simulink model "Roll_Reduced_Model_R2023b"  (R2023b)
settings: Solver=VariableStepAuto  StartTime=0.0  StopTime=10.0  RelTol=1e-3
PreLoadFcn:
  | MyParameters
values from neighbouring files (symbols this model uses):
  b = 0    [MyParameters.m]
  CurrThrust = 50    [MyParameters.m]
  g = 9.81    [MyParameters.m]
  Jpitch = 0.076089    [MyParameters.m]
  Jroll = 0.0520129    [MyParameters.m]
  Lp = 0.24    [MyParameters.m]
  Lr = 0.24    [MyParameters.m]
  mp = 2.464    [MyParameters.m]
  mr = 2    [MyParameters.m]
  rp = 0.107654    [MyParameters.m]
  rr = 0.072538    [MyParameters.m]
libraries: slpidlib x4, simulink x2
settings Model: Creator=user  LastModifiedBy=user
settings SolverCC: AlgebraicLoopSolver=TrustRegion

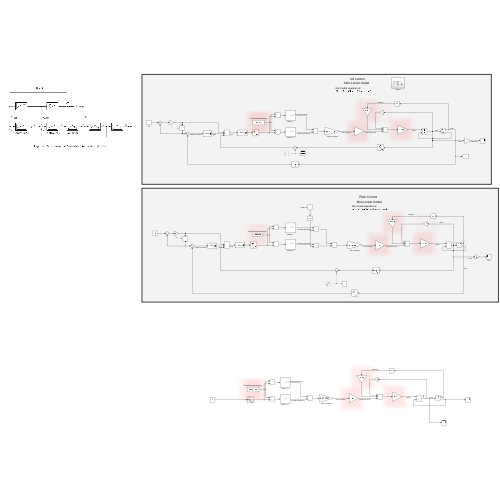
[thumbnail: Simulink's stored preview of the top-level diagram]
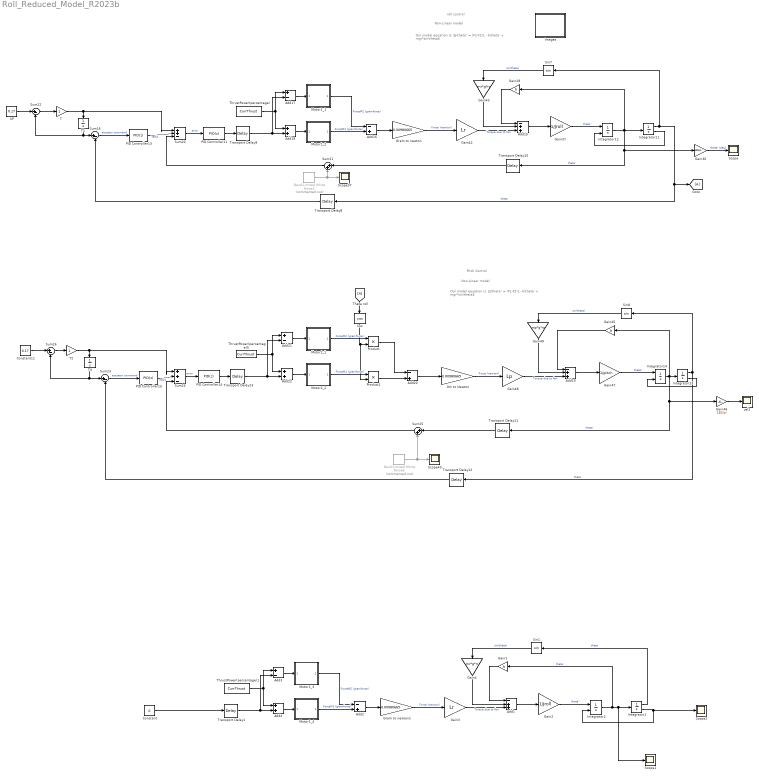
== system Roll_Reduced_Model_R2023b ==
  note: Our model equation is:
      | $J\theta'' = (F1-F2)L - b\theta' + mgr*sin\theta$
  note: Our model equation is:
      | $J\theta'' = (F1-F2)L - b\theta' + mgr*sin\theta$
  note: Non-Linear model
  note: Pitch Control
  note: Non-Linear model
  note: roll control
  Add1 : Sum  Inputs=-++
  Add15 : Sum  Inputs=-++
  Add16 : Sum  Inputs=-+
  Add17 : Sum  Inputs=+-
  Add18 : Sum
  Add19 : Sum  Inputs=-++
  Add2 : Sum  Inputs=-+
  Add20 : Sum  Inputs=-+
  Add21 : Sum  Inputs=+-
  Add22 : Sum
  Add3 : Sum  Inputs=+-
  Add4 : Sum
  Band-Limited White Noise3 : simulink/Sources/Band-Limited White Noise  Commented=on  Cov=0.000005  Ts=0.0225  seed=[23341]
  Band-Limited White Noise5 : simulink/Sources/Band-Limited White Noise  Commented=on  Cov=0.000005  Ts=0.0225  seed=[23341]
  Constant : Constant  Value=0
  Constant11 : Constant  Value=0.17
  Cos : Trigonometry  Operator=cos
  Gain1 : Gain  Gain=b
  Gain2 : Gain  Gain=1/Jroll
  Gain28 : Gain  Gain=b
  Gain3 : Gain  Gain=Lr
  Gain36 : Gain  Gain=180/pi
  Gain37 : Gain  Gain=1/Jroll
  Gain4 : Gain  Gain=mr*g*rr
  Gain42 : Gain  Gain=Lr
  Gain43 : Gain  Gain=mr*g*rr
  Gain45 : Gain  Gain=b
  Gain46 : Gain  Gain=180/pi
  Gain47 : Gain  Gain=1/Jpitch
  Gain48 : Gain  Gain=Lp
  Gain49 : Gain  Gain=mp*g*rp
  Gm to Newton : Gain  Gain=0.00980665
  Goto : Goto
  Gram to newton : Gain  Gain=0.00980665
  Gram to newton1 : Gain  Gain=0.00980665
  Images : Subsystem
  Integrator1 : Integrator  LimitOutput=on  UpperSaturationLimit=0.7  LowerSaturationLimit=-0.7  ShowSaturationPort=on
  Integrator11 : Integrator  LimitOutput=on  UpperSaturationLimit=0.7  LowerSaturationLimit=-0.7  ShowSaturationPort=on
  Integrator12 : Integrator  ExternalReset=level hold
  Integrator13 : Integrator  LimitOutput=on  UpperSaturationLimit=0.7  LowerSaturationLimit=-0.7  ShowSaturationPort=on
  Integrator14 : Integrator  ExternalReset=level hold
  Integrator2 : Integrator  ExternalReset=level hold
  Motor1_1 : Subsystem
      mask Display: image('2200kv.jpg');
  Motor1_2 : Subsystem
      mask Display: image('2200kv.jpg');
  Motor1_3 : Subsystem
      mask Display: image('2200kv.jpg');
  Motor1_4 : Subsystem
      mask Display: image('2200kv.jpg');
  Motor2_1 : Subsystem
      mask Display: image('2200kv.jpg');
  Motor2_2 : Subsystem
      mask Display: image('2200kv.jpg');
  PID Controller11 : slpidlib/PID Controller  Controller=PID  Form=Parallel  TimeDomain=Discrete-time  UseExternalTs=off  SampleTime=0.005  IntegratorMethod=Forward Euler  FilterMethod=Forward Euler  ControllerParametersSource=internal  P=4.5  I=60  UseKiTs=off  D=1.2  N=10  UseFilter=on  TunerSelectOption=Transfer Function Based (PID Tuner App)  InitialConditionSource=internal  InitialConditionForIntegrator=0  InitialConditionForFilter=0  DifferentiatorICPrevScaledInput=0  ExternalReset=none  TrackingMode=off  Kt=1  LimitOutput=on  SatLimitsSource=internal  UpperSaturationLimit=40  LowerSaturationLimit=-40  LinearizeAsGain=on  AntiWindupMode=clamping  Kb=1  LimitIntegrator=off  UpperIntegratorSaturationLimit=inf  LowerIntegratorSaturationLimit=-inf  POutMin=[]  POutMax=[]  IOutMin=[]  IOutMax=[]  DOutMin=[]  DOutMax=[]  NOutMin=[]  NOutMax=[]  SumOutMin=[]  SumOutMax=[]  SaturationOutMin=[]  SaturationOutMax=[]  PParamMin=[]  PParamMax=[]  IParamMin=[]  IParamMax=[]  DParamMin=[]  DParamMax=[]  NParamMin=[]  NParamMax=[]  KbParamMin=[]  KbParamMax=[]  KtParamMin=[]  KtParamMax=[]  KbOutMin=[]  KbOutMax=[]  KtOutMin=[]  KtOutMax=[]  IntegratorOutMin=[]  IntegratorOutMax=[]  FilterOutMin=[]  FilterOutMax=[]  SumI1OutMin=[]  SumI1OutMax=[]  SumI2OutMin=[]  SumI2OutMax=[]  SumI3OutMin=[]  SumI3OutMax=[]  SumI4OutMin=[]  SumI4OutMax=[]  SumDOutMin=[]  SumDOutMax=[]  DifferentiatorOutMin=[]  DifferentiatorOutMax=[]  FilterDiffOutCoefMin=[]  FilterDiffOutCoefMax=[]  ReciprocalOutMin=[]  ReciprocalOutMax=[]  SumDenOutMin=[]  SumDenOutMax=[]  SumNumOutMin=[]  SumNumOutMax=[]  DivideOutMin=[]  DivideOutMax=[]  UdiffTsProdOutMin=[]  UdiffTsProdOutMax=[]  NTsProdOutMin=[]  NTsProdOutMax=[]  UintegralTsProdOutMin=[]  UintegralTsProdOutMax=[]  UngainTsProdOutMin=[]  UngainTsProdOutMax=[]  ClampingZeroOutDataTypeStr=Inherit: Inherit via back propagation  ClampingZeroOutMin=[]  ClampingZeroOutMax=[]  FilterDenConstantOutDataTypeStr=Inherit: Inherit via back propagation  FilterDenConstantOutMin=[]  FilterDenConstantOutMax=[]  PCopyOutDataTypeStr=Inherit: Inherit via back propagation  PCopyOutMin=[]  PCopyOutMax=[]  NCopyOutDataTypeStr=Inherit: Inherit via back propagation  NCopyOutMin=[]  NCopyOutMax=[]  IntegratorContinuousStateAttributes=''  IntegratorStateMustResolveToSignalObject=off  IntegratorRTWStateStorageClass=Auto  FilterContinuousStateAttributes=''  FilterStateMustResolveToSignalObject=off  FilterRTWStateStorageClass=Auto  ParallelPVariant=InternalParameters  IdealPVariant=Disabled  IVariant=InternalParameters  DVariant=InternalParameters  IntegratorVariant=Discrete  SatVariant=Enabled  AWVariant=DiscClampingParallel  PCopyVariant=Disabled  TRVariant=Disabled  FdbkBlocksVariant=Forward  IdealPFdbkVariant=Disabled  SatFdbkVariant=Disabled  DerivativeFilterVariant=ForwardEulerFilter  NVariant=InternalParameters  NCopyVariant=Disabled  FilterICVariant=InternalICsFilter  IntegratorICVariant=InternalICs  ExternalResetVariant=Disabled  TRSumVariant=Passthrough  SumFdbkVariant=Disabled  SumVariant=Sum_PID  TsampFilterVariant=InternalTs  TsampNgainVariant=Passthrough  TsampIntegralVariant=Disabled_SignalSpec  ExternalSaturationOutDataTypeStr=Inherit: Same as second input
  PID Controller13 : slpidlib/PID Controller  Controller=PID  Form=Parallel  TimeDomain=Discrete-time  UseExternalTs=off  SampleTime=0.005  IntegratorMethod=Forward Euler  FilterMethod=Forward Euler  ControllerParametersSource=internal  P=1.2  I=0  UseKiTs=off  D=0  N=100  UseFilter=on  TunerSelectOption=Transfer Function Based (PID Tuner App)  InitialConditionSource=internal  InitialConditionForIntegrator=0  InitialConditionForFilter=0  DifferentiatorICPrevScaledInput=0  ExternalReset=none  TrackingMode=off  Kt=1  LimitOutput=on  SatLimitsSource=internal  UpperSaturationLimit=30  LowerSaturationLimit=-30  LinearizeAsGain=on  AntiWindupMode=clamping  Kb=1  LimitIntegrator=off  UpperIntegratorSaturationLimit=inf  LowerIntegratorSaturationLimit=-inf  POutMin=[]  POutMax=[]  IOutMin=[]  IOutMax=[]  DOutMin=[]  DOutMax=[]  NOutMin=[]  NOutMax=[]  SumOutMin=[]  SumOutMax=[]  SaturationOutMin=[]  SaturationOutMax=[]  PParamMin=[]  PParamMax=[]  IParamMin=[]  IParamMax=[]  DParamMin=[]  DParamMax=[]  NParamMin=[]  NParamMax=[]  KbParamMin=[]  KbParamMax=[]  KtParamMin=[]  KtParamMax=[]  KbOutMin=[]  KbOutMax=[]  KtOutMin=[]  KtOutMax=[]  IntegratorOutMin=[]  IntegratorOutMax=[]  FilterOutMin=[]  FilterOutMax=[]  SumI1OutMin=[]  SumI1OutMax=[]  SumI2OutMin=[]  SumI2OutMax=[]  SumI3OutMin=[]  SumI3OutMax=[]  SumI4OutMin=[]  SumI4OutMax=[]  SumDOutMin=[]  SumDOutMax=[]  DifferentiatorOutMin=[]  DifferentiatorOutMax=[]  FilterDiffOutCoefMin=[]  FilterDiffOutCoefMax=[]  ReciprocalOutMin=[]  ReciprocalOutMax=[]  SumDenOutMin=[]  SumDenOutMax=[]  SumNumOutMin=[]  SumNumOutMax=[]  DivideOutMin=[]  DivideOutMax=[]  UdiffTsProdOutMin=[]  UdiffTsProdOutMax=[]  NTsProdOutMin=[]  NTsProdOutMax=[]  UintegralTsProdOutMin=[]  UintegralTsProdOutMax=[]  UngainTsProdOutMin=[]  UngainTsProdOutMax=[]  ClampingZeroOutDataTypeStr=Inherit: Inherit via back propagation  ClampingZeroOutMin=[]  ClampingZeroOutMax=[]  FilterDenConstantOutDataTypeStr=Inherit: Inherit via back propagation  FilterDenConstantOutMin=[]  FilterDenConstantOutMax=[]  PCopyOutDataTypeStr=Inherit: Inherit via back propagation  PCopyOutMin=[]  PCopyOutMax=[]  NCopyOutDataTypeStr=Inherit: Inherit via back propagation  NCopyOutMin=[]  NCopyOutMax=[]  IntegratorContinuousStateAttributes=''  IntegratorStateMustResolveToSignalObject=off  IntegratorRTWStateStorageClass=Auto  FilterContinuousStateAttributes=''  FilterStateMustResolveToSignalObject=off  FilterRTWStateStorageClass=Auto  ParallelPVariant=InternalParameters  IdealPVariant=Disabled  IVariant=InternalParameters  DVariant=InternalParameters  IntegratorVariant=Discrete  SatVariant=Enabled  AWVariant=DiscClampingParallel  PCopyVariant=Disabled  TRVariant=Disabled  FdbkBlocksVariant=Forward  IdealPFdbkVariant=Disabled  SatFdbkVariant=Disabled  DerivativeFilterVariant=ForwardEulerFilter  NVariant=InternalParameters  NCopyVariant=Disabled  FilterICVariant=InternalICsFilter  IntegratorICVariant=InternalICs  ExternalResetVariant=Disabled  TRSumVariant=Passthrough  SumFdbkVariant=Disabled  SumVariant=Sum_PID  TsampFilterVariant=InternalTs  TsampNgainVariant=Passthrough  TsampIntegralVariant=Disabled_SignalSpec  ExternalSaturationOutDataTypeStr=Inherit: Same as second input
  PID Controller14 : slpidlib/PID Controller  Controller=PID  Form=Parallel  TimeDomain=Discrete-time  UseExternalTs=off  SampleTime=0.005  IntegratorMethod=Forward Euler  FilterMethod=Forward Euler  ControllerParametersSource=internal  P=9  I=60  UseKiTs=off  D=1.2  N=10  UseFilter=on  TunerSelectOption=Transfer Function Based (PID Tuner App)  InitialConditionSource=internal  InitialConditionForIntegrator=0  InitialConditionForFilter=0  DifferentiatorICPrevScaledInput=0  ExternalReset=none  TrackingMode=off  Kt=1  LimitOutput=on  SatLimitsSource=internal  UpperSaturationLimit=40  LowerSaturationLimit=-40  LinearizeAsGain=on  AntiWindupMode=clamping  Kb=1  LimitIntegrator=off  UpperIntegratorSaturationLimit=inf  LowerIntegratorSaturationLimit=-inf  POutMin=[]  POutMax=[]  IOutMin=[]  IOutMax=[]  DOutMin=[]  DOutMax=[]  NOutMin=[]  NOutMax=[]  SumOutMin=[]  SumOutMax=[]  SaturationOutMin=[]  SaturationOutMax=[]  PParamMin=[]  PParamMax=[]  IParamMin=[]  IParamMax=[]  DParamMin=[]  DParamMax=[]  NParamMin=[]  NParamMax=[]  KbParamMin=[]  KbParamMax=[]  KtParamMin=[]  KtParamMax=[]  KbOutMin=[]  KbOutMax=[]  KtOutMin=[]  KtOutMax=[]  IntegratorOutMin=[]  IntegratorOutMax=[]  FilterOutMin=[]  FilterOutMax=[]  SumI1OutMin=[]  SumI1OutMax=[]  SumI2OutMin=[]  SumI2OutMax=[]  SumI3OutMin=[]  SumI3OutMax=[]  SumI4OutMin=[]  SumI4OutMax=[]  SumDOutMin=[]  SumDOutMax=[]  DifferentiatorOutMin=[]  DifferentiatorOutMax=[]  FilterDiffOutCoefMin=[]  FilterDiffOutCoefMax=[]  ReciprocalOutMin=[]  ReciprocalOutMax=[]  SumDenOutMin=[]  SumDenOutMax=[]  SumNumOutMin=[]  SumNumOutMax=[]  DivideOutMin=[]  DivideOutMax=[]  UdiffTsProdOutMin=[]  UdiffTsProdOutMax=[]  NTsProdOutMin=[]  NTsProdOutMax=[]  UintegralTsProdOutMin=[]  UintegralTsProdOutMax=[]  UngainTsProdOutMin=[]  UngainTsProdOutMax=[]  ClampingZeroOutDataTypeStr=Inherit: Inherit via back propagation  ClampingZeroOutMin=[]  ClampingZeroOutMax=[]  FilterDenConstantOutDataTypeStr=Inherit: Inherit via back propagation  FilterDenConstantOutMin=[]  FilterDenConstantOutMax=[]  PCopyOutDataTypeStr=Inherit: Inherit via back propagation  PCopyOutMin=[]  PCopyOutMax=[]  NCopyOutDataTypeStr=Inherit: Inherit via back propagation  NCopyOutMin=[]  NCopyOutMax=[]  IntegratorContinuousStateAttributes=''  IntegratorStateMustResolveToSignalObject=off  IntegratorRTWStateStorageClass=Auto  FilterContinuousStateAttributes=''  FilterStateMustResolveToSignalObject=off  FilterRTWStateStorageClass=Auto  ParallelPVariant=InternalParameters  IdealPVariant=Disabled  IVariant=InternalParameters  DVariant=InternalParameters  IntegratorVariant=Discrete  SatVariant=Enabled  AWVariant=DiscClampingParallel  PCopyVariant=Disabled  TRVariant=Disabled  FdbkBlocksVariant=Forward  IdealPFdbkVariant=Disabled  SatFdbkVariant=Disabled  DerivativeFilterVariant=ForwardEulerFilter  NVariant=InternalParameters  NCopyVariant=Disabled  FilterICVariant=InternalICsFilter  IntegratorICVariant=InternalICs  ExternalResetVariant=Disabled  TRSumVariant=Passthrough  SumFdbkVariant=Disabled  SumVariant=Sum_PID  TsampFilterVariant=InternalTs  TsampNgainVariant=Passthrough  TsampIntegralVariant=Disabled_SignalSpec  ExternalSaturationOutDataTypeStr=Inherit: Same as second input
  PID Controller15 : slpidlib/PID Controller  Controller=PID  Form=Parallel  TimeDomain=Discrete-time  UseExternalTs=off  SampleTime=0.005  IntegratorMethod=Forward Euler  FilterMethod=Forward Euler  ControllerParametersSource=internal  P=1.5  I=0  UseKiTs=off  D=0  N=100  UseFilter=on  TunerSelectOption=Transfer Function Based (PID Tuner App)  InitialConditionSource=internal  InitialConditionForIntegrator=0  InitialConditionForFilter=0  DifferentiatorICPrevScaledInput=0  ExternalReset=none  TrackingMode=off  Kt=1  LimitOutput=on  SatLimitsSource=internal  UpperSaturationLimit=30  LowerSaturationLimit=-30  LinearizeAsGain=on  AntiWindupMode=clamping  Kb=1  LimitIntegrator=off  UpperIntegratorSaturationLimit=inf  LowerIntegratorSaturationLimit=-inf  POutMin=[]  POutMax=[]  IOutMin=[]  IOutMax=[]  DOutMin=[]  DOutMax=[]  NOutMin=[]  NOutMax=[]  SumOutMin=[]  SumOutMax=[]  SaturationOutMin=[]  SaturationOutMax=[]  PParamMin=[]  PParamMax=[]  IParamMin=[]  IParamMax=[]  DParamMin=[]  DParamMax=[]  NParamMin=[]  NParamMax=[]  KbParamMin=[]  KbParamMax=[]  KtParamMin=[]  KtParamMax=[]  KbOutMin=[]  KbOutMax=[]  KtOutMin=[]  KtOutMax=[]  IntegratorOutMin=[]  IntegratorOutMax=[]  FilterOutMin=[]  FilterOutMax=[]  SumI1OutMin=[]  SumI1OutMax=[]  SumI2OutMin=[]  SumI2OutMax=[]  SumI3OutMin=[]  SumI3OutMax=[]  SumI4OutMin=[]  SumI4OutMax=[]  SumDOutMin=[]  SumDOutMax=[]  DifferentiatorOutMin=[]  DifferentiatorOutMax=[]  FilterDiffOutCoefMin=[]  FilterDiffOutCoefMax=[]  ReciprocalOutMin=[]  ReciprocalOutMax=[]  SumDenOutMin=[]  SumDenOutMax=[]  SumNumOutMin=[]  SumNumOutMax=[]  DivideOutMin=[]  DivideOutMax=[]  UdiffTsProdOutMin=[]  UdiffTsProdOutMax=[]  NTsProdOutMin=[]  NTsProdOutMax=[]  UintegralTsProdOutMin=[]  UintegralTsProdOutMax=[]  UngainTsProdOutMin=[]  UngainTsProdOutMax=[]  ClampingZeroOutDataTypeStr=Inherit: Inherit via back propagation  ClampingZeroOutMin=[]  ClampingZeroOutMax=[]  FilterDenConstantOutDataTypeStr=Inherit: Inherit via back propagation  FilterDenConstantOutMin=[]  FilterDenConstantOutMax=[]  PCopyOutDataTypeStr=Inherit: Inherit via back propagation  PCopyOutMin=[]  PCopyOutMax=[]  NCopyOutDataTypeStr=Inherit: Inherit via back propagation  NCopyOutMin=[]  NCopyOutMax=[]  IntegratorContinuousStateAttributes=''  IntegratorStateMustResolveToSignalObject=off  IntegratorRTWStateStorageClass=Auto  FilterContinuousStateAttributes=''  FilterStateMustResolveToSignalObject=off  FilterRTWStateStorageClass=Auto  ParallelPVariant=InternalParameters  IdealPVariant=Disabled  IVariant=InternalParameters  DVariant=InternalParameters  IntegratorVariant=Discrete  SatVariant=Enabled  AWVariant=DiscClampingParallel  PCopyVariant=Disabled  TRVariant=Disabled  FdbkBlocksVariant=Forward  IdealPFdbkVariant=Disabled  SatFdbkVariant=Disabled  DerivativeFilterVariant=ForwardEulerFilter  NVariant=InternalParameters  NCopyVariant=Disabled  FilterICVariant=InternalICsFilter  IntegratorICVariant=InternalICs  ExternalResetVariant=Disabled  TRSumVariant=Passthrough  SumFdbkVariant=Disabled  SumVariant=Sum_PID  TsampFilterVariant=InternalTs  TsampNgainVariant=Passthrough  TsampIntegralVariant=Disabled_SignalSpec  ExternalSaturationOutDataTypeStr=Inherit: Same as second input
  Product : Product
  Product1 : Product
  SP : Constant  Value=0.17
  Scope{,1..2,37,43} (5 alike) : Scope
  Sin1 : Trigonometry
  Sin7 : Trigonometry
  Sin8 : Trigonometry
  Sum{16,22..23,26} (4 alike) : Sum  Inputs=|+-
  Sum20 : Sum  Inputs=|++-
  Sum21 : Sum  Inputs=|++
  Sum24 : Sum  Inputs=|++-
  Sum25 : Sum  Inputs=|++
  T : Gain
  T1 : Integrator
  T2 : Gain
  T3 : Integrator
  Theta roll : From
  ThrustPower(percentage) : Constant  Value=CurrThrust
  ThrustPower(percentage)1 : Constant  Value=CurrThrust
  ThrustPower(percentage)5 : Constant  Value=CurrThrust
  Transport Delay1 : TransportDelay  DelayTime=0.05
  Transport Delay{8,10..12} (4 alike) : TransportDelay  DelayTime=0.0225
  Transport Delay13 : TransportDelay  DelayTime=0.05
  Transport Delay9 : TransportDelay  DelayTime=0.05
  vel2 : Scope
  wires:
  Cos/1 -> Product1/2, Product/2
  Add19/1 -> Gain47/1
  ThrustPower(percentage)5/1 -> Add22/1, Add21/1
  Product1/1 -> Add20/2
  Gain49/1 -> Add19/2
  Gain45/1 -> Add19/1
  Gain37/1 -> Integrator12/1  "theta''"
  Integrator11/1 -> Transport Delay8/1, Goto/1, Sin7/1  "theta"
  Sum25/1 -> Sum24/3
  Sum24/1 -> PID Controller14/1  "error"
  Integrator14/1 -> Integrator13/1, Gain46/1, Transport Delay11/1, Gain45/1  "theta'"
  Band-Limited White Noise5/1 -> Scope43/1, Sum25/2
  Gm to Newton/1 -> Gain48/1  "Force (newton)"
  Add16/1 -> Gram to newton/1
  Gain48/1 -> Add19/3  "Torque due to fan"
  PID Controller15/1 -> Sum24/2  "rad/s"
  Motor1_1/1(MotorForce) -> Add16/1  "ForceM2 (gramforce)"
  Integrator13/1 -> Transport Delay12/1, Sin8/1  "theta"
  Add20/1 -> Gm to Newton/1
  Motor2_1/1(MotorForce) -> Product/1  "ForceM2 (gramforce)"
  Gain47/1 -> Integrator14/1  "theta''"
  Add21/1 -> Motor2_1/1(MotorPercentage)
  Gain46/1 -> vel2/1
  PID Controller11/1 -> Transport Delay9/1
  Product/1 -> Add20/1
  ThrustPower(percentage)/1 -> Add18/1, Add17/1
  Transport Delay12/1 -> Sum23/2
  Transport Delay10/1 -> Sum21/1
  Motor1_2/1(MotorForce) -> Add16/2  "ForceM1 (gramforce)"
  Motor2_2/1(MotorForce) -> Product1/1  "ForceM1 (gramforce)"
  Sum21/1 -> Sum20/3
  Add18/1 -> Motor1_2/1(MotorPercentage)
  Sum26/1 -> T2/1
  Transport Delay13/1 -> Add22/2, Add21/2
  Sum23/1 -> PID Controller15/1  "actuator command"
  Sum22/1 -> T/1
  Add22/1 -> Motor2_2/1(MotorPercentage)
  T3/1 -> Sum23/1, Sum26/2
  T/1 -> T1/1, Sum20/1
  T2/1 -> Sum24/1, T3/1
  SP/1 -> Sum22/1
  Transport Delay11/1 -> Sum25/1
  PID Controller13/1 -> Sum20/2  "rad/s"
  Sin7/1 -> Gain43/1  "sin(theta)"
  Gram to newton/1 -> Gain42/1  "Force (newton)"
  Gain42/1 -> Add15/3  "Torque due to fan"
  Add17/1 -> Motor1_1/1(MotorPercentage)
  Gain28/1 -> Add15/1
  Gain43/1 -> Add15/2
  Transport Delay8/1 -> Sum16/2
  Add15/1 -> Gain37/1
  Integrator13/2 -> Integrator14/2
  Sum20/1 -> PID Controller11/1  "error"
  Band-Limited White Noise3/1 -> Sum21/2, Scope37/1
  Transport Delay9/1 -> Add17/2, Add18/2
  T1/1 -> Sum22/2, Sum16/1
  Integrator12/1 -> Integrator11/1, Transport Delay10/1, Gain36/1, Gain28/1  "theta'"
  Sum16/1 -> PID Controller13/1  "actuator command"
  Constant11/1 -> Sum26/1
  PID Controller14/1 -> Transport Delay13/1
  Integrator11/2 -> Integrator12/2
  Sin8/1 -> Gain49/1  "sin(theta)"
  Gain36/1 -> Scope/1  "theta' (deg)"
  Theta roll/1 -> Cos/1
  Integrator1/2 -> Integrator2/2, Scope2/1
  Integrator2/1 -> Gain1/1, Scope1/1, Integrator1/1  "theta'"
  Transport Delay1/1 -> Add4/2, Add3/2
  Add1/1 -> Gain2/1
  Gain4/1 -> Add1/2
  Gain1/1 -> Add1/1
  Add3/1 -> Motor1_3/1(MotorPercentage)
  Gain3/1 -> Add1/3  "Torque due to fan"
  Gram to newton1/1 -> Gain3/1  "Force (newton)"
  Sin1/1 -> Gain4/1  "sin(theta)"
  Add4/1 -> Motor1_4/1(MotorPercentage)
  Motor1_4/1(MotorForce) -> Add2/2  "ForceM1 (gramforce)"
  ThrustPower(percentage)1/1 -> Add3/1, Add4/1
  Motor1_3/1(MotorForce) -> Add2/1  "ForceM2 (gramforce)"
  Add2/1 -> Gram to newton1/1
  Integrator1/1 -> Sin1/1  "theta"
  Gain2/1 -> Integrator2/1  "theta''"
  Constant/1 -> Transport Delay1/1

== system Roll_Reduced_Model_R2023b/Images ==

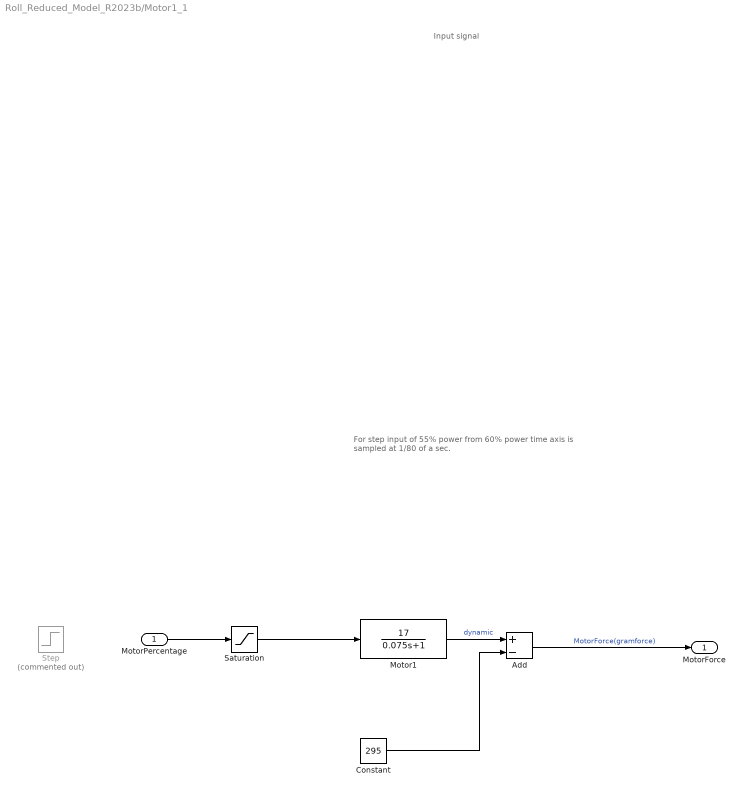
== system Roll_Reduced_Model_R2023b/Motor1_1 ==
  note: Input signal
  note: For step input of 55% power from 60% power
      | time axis is sampled at 1/80 of a sec.
  MotorPercentage : Inport
  Add : Sum  Inputs=+-
  Constant : Constant  Value=295
  Motor1 : TransferFcn  Numerator=[17]  Denominator=[0.075 1]
  Saturation : Saturate  UpperLimit=100  LowerLimit=0
  Step : Step  Commented=on  Time=2  Before=60  After=55  SampleTime=0
  MotorForce : Outport
  wires:
  Saturation/1 -> Motor1/1
  MotorPercentage/1 -> Saturation/1
  Add/1 -> MotorForce/1  "MotorForce(gramforce)"
  Motor1/1 -> Add/1  "dynamic"
  Constant/1 -> Add/2

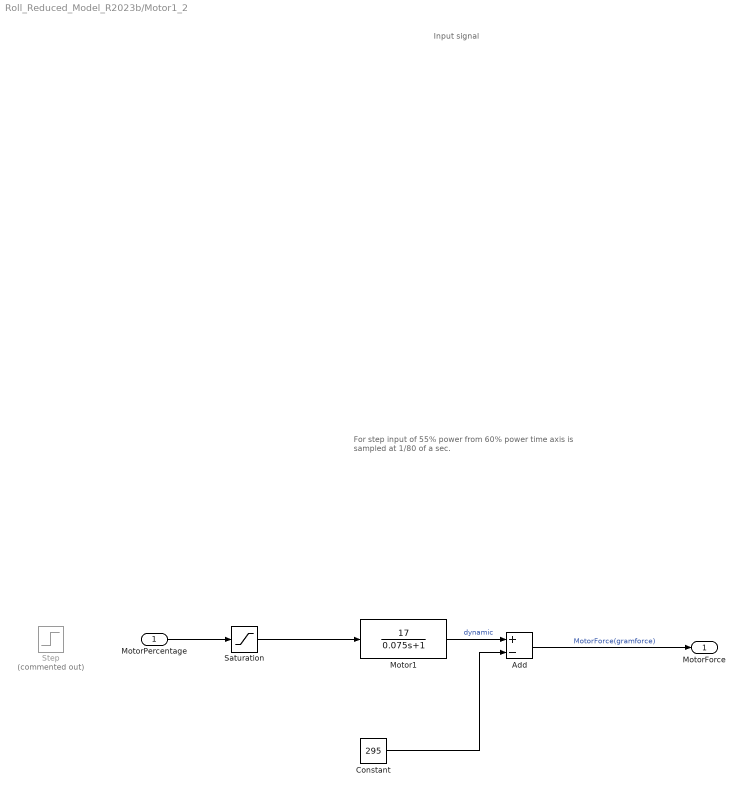
== system Roll_Reduced_Model_R2023b/Motor1_2 ==
  note: For step input of 55% power from 60% power
      | time axis is sampled at 1/80 of a sec.
  note: Input signal
  MotorPercentage : Inport
  Add : Sum  Inputs=+-
  Constant : Constant  Value=295
  Motor1 : TransferFcn  Numerator=[17]  Denominator=[0.075 1]
  Saturation : Saturate  UpperLimit=100  LowerLimit=0
  Step : Step  Commented=on  Time=2  Before=60  After=55  SampleTime=0
  MotorForce : Outport
  wires:
  Constant/1 -> Add/2
  Motor1/1 -> Add/1  "dynamic"
  Add/1 -> MotorForce/1  "MotorForce(gramforce)"
  MotorPercentage/1 -> Saturation/1
  Saturation/1 -> Motor1/1

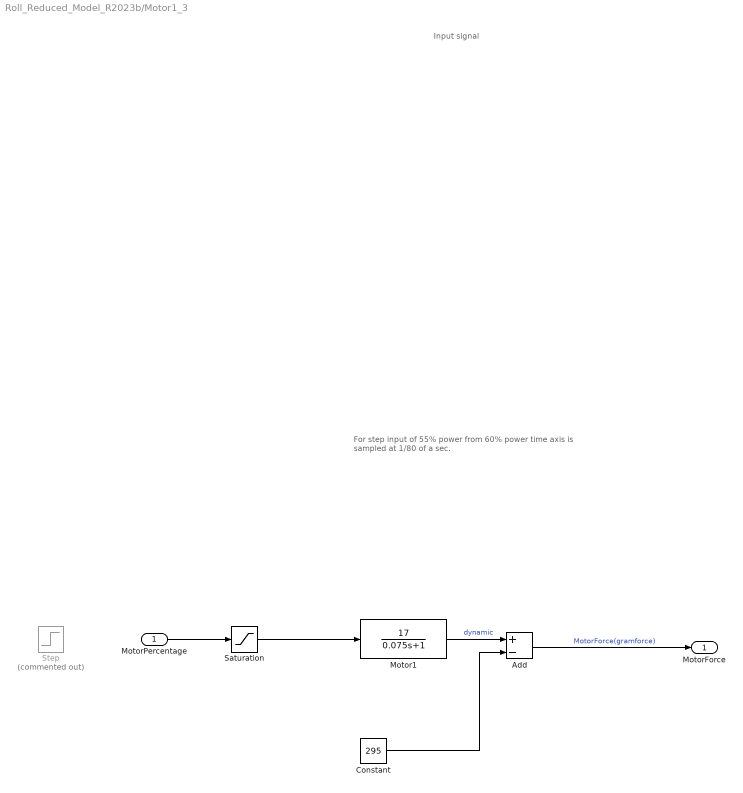
== system Roll_Reduced_Model_R2023b/Motor1_3 ==
  note: For step input of 55% power from 60% power
      | time axis is sampled at 1/80 of a sec.
  note: Input signal
  MotorPercentage : Inport
  Add : Sum  Inputs=+-
  Constant : Constant  Value=295
  Motor1 : TransferFcn  Numerator=[17]  Denominator=[0.075 1]
  Saturation : Saturate  UpperLimit=100  LowerLimit=0
  Step : Step  Commented=on  Time=2  Before=60  After=55  SampleTime=0
  MotorForce : Outport
  wires:
  Constant/1 -> Add/2
  Motor1/1 -> Add/1  "dynamic"
  Add/1 -> MotorForce/1  "MotorForce(gramforce)"
  MotorPercentage/1 -> Saturation/1
  Saturation/1 -> Motor1/1

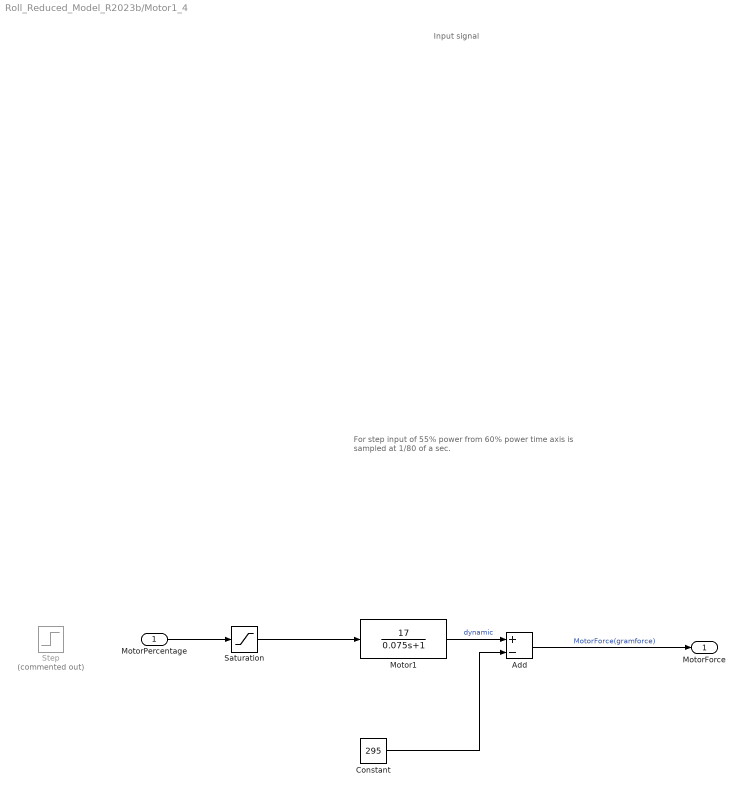
== system Roll_Reduced_Model_R2023b/Motor1_4 ==
  note: Input signal
  note: For step input of 55% power from 60% power
      | time axis is sampled at 1/80 of a sec.
  MotorPercentage : Inport
  Add : Sum  Inputs=+-
  Constant : Constant  Value=295
  Motor1 : TransferFcn  Numerator=[17]  Denominator=[0.075 1]
  Saturation : Saturate  UpperLimit=100  LowerLimit=0
  Step : Step  Commented=on  Time=2  Before=60  After=55  SampleTime=0
  MotorForce : Outport
  wires:
  Saturation/1 -> Motor1/1
  MotorPercentage/1 -> Saturation/1
  Add/1 -> MotorForce/1  "MotorForce(gramforce)"
  Motor1/1 -> Add/1  "dynamic"
  Constant/1 -> Add/2

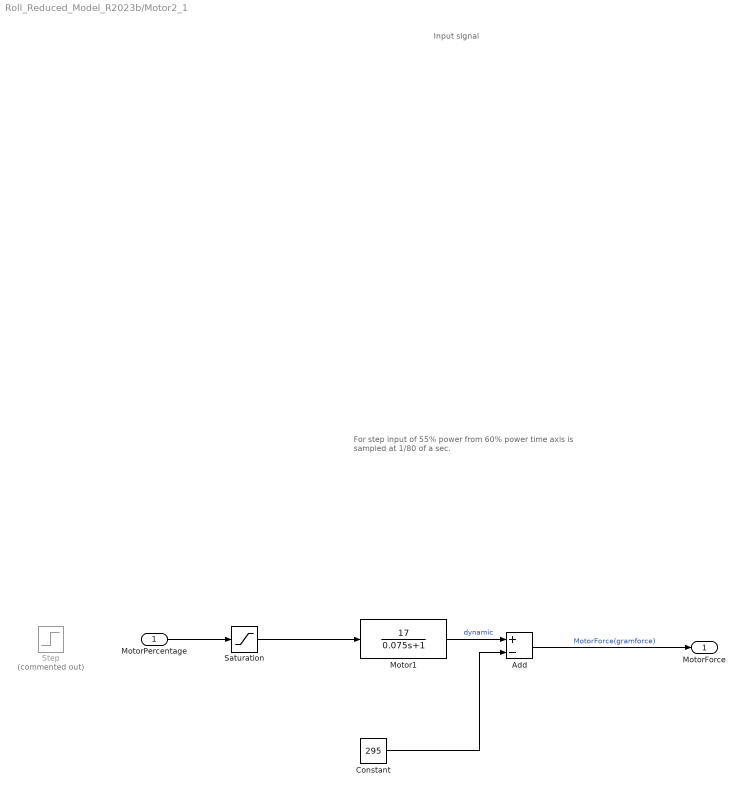
== system Roll_Reduced_Model_R2023b/Motor2_1 ==
  note: For step input of 55% power from 60% power
      | time axis is sampled at 1/80 of a sec.
  note: Input signal
  MotorPercentage : Inport
  Add : Sum  Inputs=+-
  Constant : Constant  Value=295
  Motor1 : TransferFcn  Numerator=[17]  Denominator=[0.075 1]
  Saturation : Saturate  UpperLimit=100  LowerLimit=0
  Step : Step  Commented=on  Time=2  Before=60  After=55  SampleTime=0
  MotorForce : Outport
  wires:
  Constant/1 -> Add/2
  Motor1/1 -> Add/1  "dynamic"
  Add/1 -> MotorForce/1  "MotorForce(gramforce)"
  MotorPercentage/1 -> Saturation/1
  Saturation/1 -> Motor1/1

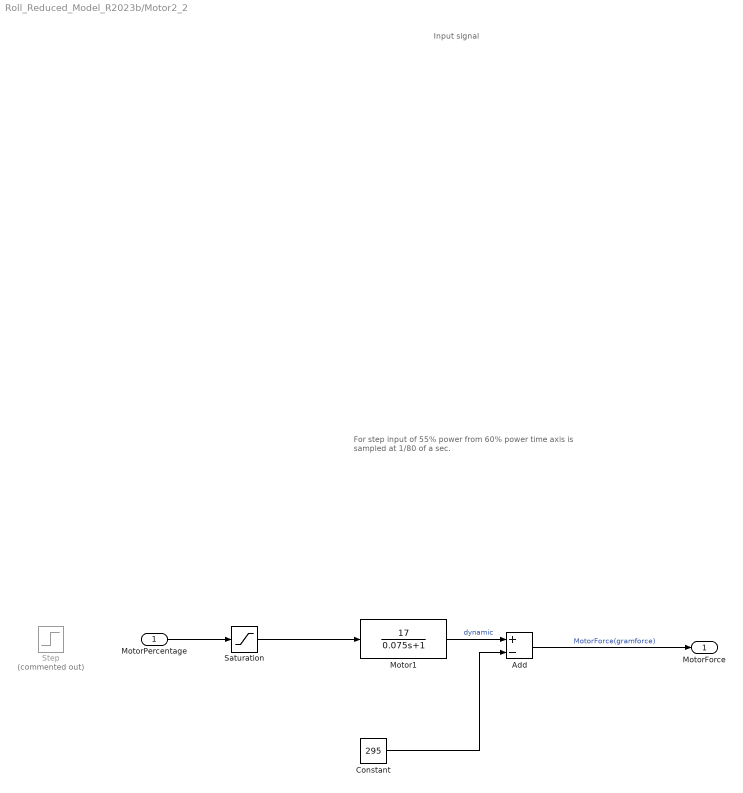
== system Roll_Reduced_Model_R2023b/Motor2_2 ==
  note: Input signal
  note: For step input of 55% power from 60% power
      | time axis is sampled at 1/80 of a sec.
  MotorPercentage : Inport
  Add : Sum  Inputs=+-
  Constant : Constant  Value=295
  Motor1 : TransferFcn  Numerator=[17]  Denominator=[0.075 1]
  Saturation : Saturate  UpperLimit=100  LowerLimit=0
  Step : Step  Commented=on  Time=2  Before=60  After=55  SampleTime=0
  MotorForce : Outport
  wires:
  Saturation/1 -> Motor1/1
  MotorPercentage/1 -> Saturation/1
  Add/1 -> MotorForce/1  "MotorForce(gramforce)"
  Motor1/1 -> Add/1  "dynamic"
  Constant/1 -> Add/2
